simulink model "SPMSM_speed_control_with_decoupling"  (R2023b)
settings: Solver=ode45  StartTime=0.0  StopTime=3  MaxStep=0.001  RelTol=1e-3
values from neighbouring files (symbols this model uses):
  J_motor = 0.0027    [PMSM_parameter2.m]
  Lamda = 0.1194    [PMSM_parameter2.m]
  Ld = 0.0003752    [PMSM_parameter2.m]
  Lq = 0.0003752    [PMSM_parameter2.m]
  Ls = 0.0003752    [PMSM_parameter2.m]
  Pole = 2    [PMSM_parameter2.m]
  R = 0.2    [PMSM_parameter2.m]
  T_load = 10    [PMSM_parameter2.m]
  w_base = (60/(2*pi))*(v_rated/sqrt((Ls^2)*(T_load/1.5*Pole*Lamda)^2+(Lamda^2)))    [PMSM_parameter2.m]
  w_ref = 3000    [PMSM_parameter2.m]
undefined symbols (not defined in the file or in its folder): v_rated
libraries: mcbcontrolslib x2, simulink_extras x1, slpidlib x1
settings Model: Creator=chayutht  LastModifiedBy=chayutht

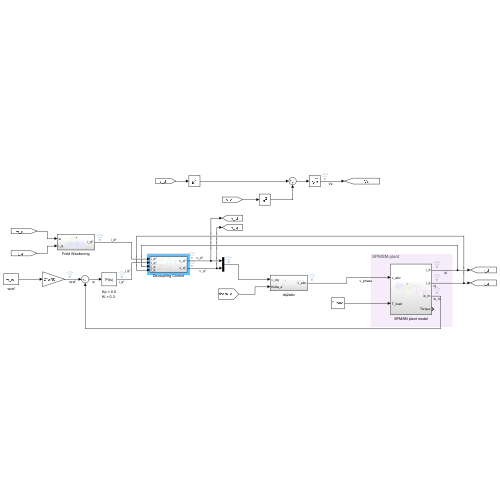
[thumbnail: Simulink's stored preview of the top-level diagram]
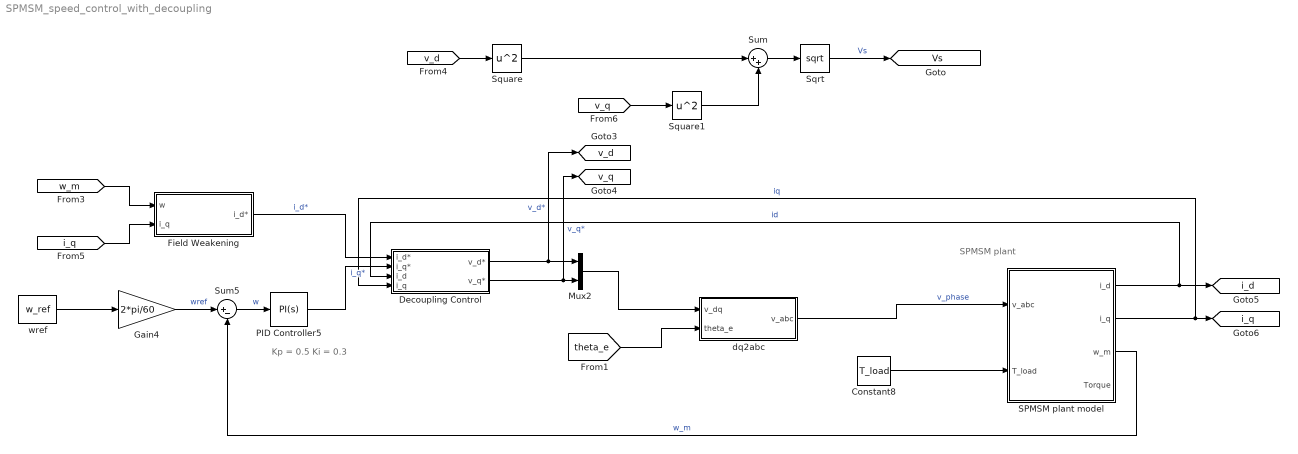
== system SPMSM_speed_control_with_decoupling ==
  note: SPMSM plant
  note: Kp = 0.5
      | Ki = 0.3
  Constant8 : Constant  Value=T_load
  Decoupling Control : Subsystem
  Field Weakening : Subsystem
  Gain4 : Gain  Gain=2*pi/60
  Mux2 : Mux  Inputs=2
  PID Controller5 : slpidlib/PID Controller  Controller=PI  Form=Parallel  TimeDomain=Continuous-time  UseExternalTs=off  SampleTime=-1  IntegratorMethod=Forward Euler  FilterMethod=Forward Euler  ControllerParametersSource=internal  P=0.2  I=0.3  UseKiTs=off  D=0  N=100  UseFilter=on  TunerSelectOption=Transfer Function Based (PID Tuner App)  InitialConditionSource=internal  InitialConditionForIntegrator=0  InitialConditionForFilter=0  DifferentiatorICPrevScaledInput=0  ExternalReset=none  TrackingMode=off  Kt=1  LimitOutput=off  SatLimitsSource=internal  UpperSaturationLimit=inf  LowerSaturationLimit=-inf  LinearizeAsGain=on  AntiWindupMode=none  Kb=1  LimitIntegrator=off  UpperIntegratorSaturationLimit=inf  LowerIntegratorSaturationLimit=-inf  POutMin=[]  POutMax=[]  IOutMin=[]  IOutMax=[]  DOutMin=[]  DOutMax=[]  NOutMin=[]  NOutMax=[]  SumOutMin=[]  SumOutMax=[]  SaturationOutMin=[]  SaturationOutMax=[]  PParamMin=[]  PParamMax=[]  IParamMin=[]  IParamMax=[]  DParamMin=[]  DParamMax=[]  NParamMin=[]  NParamMax=[]  KbParamMin=[]  KbParamMax=[]  KtParamMin=[]  KtParamMax=[]  KbOutMin=[]  KbOutMax=[]  KtOutMin=[]  KtOutMax=[]  IntegratorOutMin=[]  IntegratorOutMax=[]  FilterOutMin=[]  FilterOutMax=[]  SumI1OutMin=[]  SumI1OutMax=[]  SumI2OutMin=[]  SumI2OutMax=[]  SumI3OutMin=[]  SumI3OutMax=[]  SumI4OutMin=[]  SumI4OutMax=[]  SumDOutMin=[]  SumDOutMax=[]  DifferentiatorOutMin=[]  DifferentiatorOutMax=[]  FilterDiffOutCoefMin=[]  FilterDiffOutCoefMax=[]  ReciprocalOutMin=[]  ReciprocalOutMax=[]  SumDenOutMin=[]  SumDenOutMax=[]  SumNumOutMin=[]  SumNumOutMax=[]  DivideOutMin=[]  DivideOutMax=[]  UdiffTsProdOutMin=[]  UdiffTsProdOutMax=[]  NTsProdOutMin=[]  NTsProdOutMax=[]  UintegralTsProdOutMin=[]  UintegralTsProdOutMax=[]  UngainTsProdOutMin=[]  UngainTsProdOutMax=[]  ClampingZeroOutDataTypeStr=Inherit: Inherit via back propagation  ClampingZeroOutMin=[]  ClampingZeroOutMax=[]  FilterDenConstantOutDataTypeStr=Inherit: Inherit via back propagation  FilterDenConstantOutMin=[]  FilterDenConstantOutMax=[]  PCopyOutDataTypeStr=Inherit: Inherit via back propagation  PCopyOutMin=[]  PCopyOutMax=[]  NCopyOutDataTypeStr=Inherit: Inherit via back propagation  NCopyOutMin=[]  NCopyOutMax=[]  IntegratorContinuousStateAttributes=''  IntegratorStateMustResolveToSignalObject=off  IntegratorRTWStateStorageClass=Auto  FilterContinuousStateAttributes=''  FilterStateMustResolveToSignalObject=off  FilterRTWStateStorageClass=Auto  ParallelPVariant=InternalParameters  IdealPVariant=Disabled  IVariant=InternalParameters  DVariant=Disabled  IntegratorVariant=Continuous  SatVariant=Disabled  AWVariant=Passthrough  PCopyVariant=Disabled  TRVariant=Disabled  FdbkBlocksVariant=Forward  IdealPFdbkVariant=Disabled  SatFdbkVariant=Disabled  DerivativeFilterVariant=Disabled  NVariant=Disabled  NCopyVariant=Disabled_SignalSpec  FilterICVariant=Disabled  IntegratorICVariant=InternalICs  ExternalResetVariant=Disabled  TRSumVariant=Passthrough  SumFdbkVariant=Disabled  SumVariant=Sum_PI  TsampFilterVariant=InternalTs  TsampNgainVariant=Passthrough  TsampIntegralVariant=Disabled_SignalSpec  ExternalSaturationOutDataTypeStr=Inherit: Same as second input
  SPMSM plant model : Subsystem
  Sqrt : Sqrt
  Square : Math  Operator=square
  Square1 : Math  Operator=square
  Sum : Sum  Inputs=|++
  Sum5 : Sum  Inputs=|+-
  dq2abc : Subsystem
  wref : Constant  Value=w_ref
  tag scope: Vs=global, i_d=global, i_q=global, v_d=global, v_q=global
  wires:
  [w_m] -> Field Weakening/1(w)
  PID Controller5/1 -> Decoupling Control/2(i_q*)  "i_q*"
  Gain4/1 -> Sum5/1  "wref"
  Decoupling Control/1(v_d*) -> [v_d], Mux2/1  "v_d*"
  Mux2/1 -> dq2abc/1(v_dq)
  [i_q] -> Field Weakening/2(i_q)
  Sum5/1 -> PID Controller5/1  "w"
  SPMSM plant model/1(i_d) -> Decoupling Control/3(i_d), [i_d]  "id"
  dq2abc/1(v_abc) -> SPMSM plant model/1(v_abc)  "v_phase"
  wref/1 -> Gain4/1
  Decoupling Control/2(v_q*) -> [v_q], Mux2/2  "v_q*"
  Field Weakening/1(i_d*) -> Decoupling Control/1(i_d*)  "i_d*"
  [theta_e] -> dq2abc/2(theta_e)
  SPMSM plant model/3(w_m) -> Sum5/2  "w_m"
  Constant8/1 -> SPMSM plant model/2(T_load)
  SPMSM plant model/2(i_q) -> Decoupling Control/4(i_q), [i_q]  "iq"
  Sum/1 -> Sqrt/1
  Sqrt/1 -> [Vs]  "Vs"
  Square/1 -> Sum/1
  [v_d] -> Square/1
  Square1/1 -> Sum/2
  [v_q] -> Square1/1

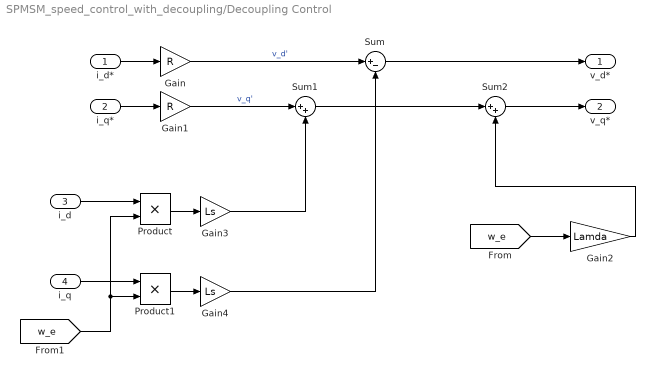
== system SPMSM_speed_control_with_decoupling/Decoupling Control ==
  i_d* : Inport
  i_q* : Inport  Port=2
  i_d : Inport  Port=3
  i_q : Inport  Port=4
  Gain : Gain  Gain=R
  Gain1 : Gain  Gain=R
  Gain2 : Gain  Gain=Lamda
  Gain3 : Gain  Gain=Ls
  Gain4 : Gain  Gain=Ls
  Product : Product
  Product1 : Product
  Sum : Sum  Inputs=|+-
  Sum1 : Sum  Inputs=|++
  Sum2 : Sum  Inputs=|++
  v_d* : Outport
  v_q* : Outport  Port=2
  wires:
  i_d*/1 -> Gain/1
  i_q*/1 -> Gain1/1
  Gain1/1 -> Sum1/1  "v_q'"
  Gain/1 -> Sum/1  "v_d'"
  Sum1/1 -> Sum2/1
  Sum2/1 -> v_q*/1
  Sum/1 -> v_d*/1
  [w_e] -> Gain2/1
  Gain2/1 -> Sum2/2
  i_d/1 -> Product/1
  [w_e] -> Product1/2, Product/2
  i_q/1 -> Product1/1
  Product/1 -> Gain3/1
  Product1/1 -> Gain4/1
  Gain3/1 -> Sum1/2
  Gain4/1 -> Sum/2

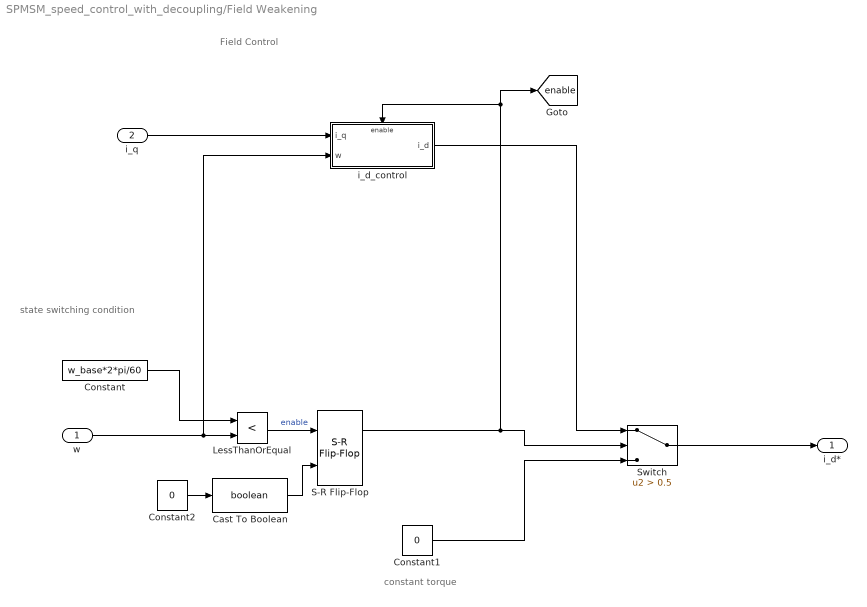
== system SPMSM_speed_control_with_decoupling/Field Weakening ==
  note: Field Control
  note: state switching condition
  note: constant torque
  w : Inport
  i_q : Inport  Port=2
  Cast To Boolean : DataTypeConversion  OutDataTypeStr=boolean  SaturateOnIntegerOverflow=off  RndMeth=Floor
  Constant : Constant  Value=w_base*2*pi/60
  Constant1 : Constant  Value=0
  Constant2 : Constant  Value=0
  LessThanOrEqual : RelationalOperator  Operator=<  OutDataTypeStr=boolean  RndMeth=Simplest  InputSameDT=off
  S-R Flip-Flop : simulink_extras/Flip Flops/S-R Flip-Flop  initial_condition=0
  Switch : Switch  Criteria=u2 > Threshold  Threshold=0.5  SaturateOnIntegerOverflow=off  InputSameDT=off
  i_d_control : Subsystem
  i_d* : Outport
  tag scope: enable=global
  wires:
  Constant/1 -> LessThanOrEqual/1
  LessThanOrEqual/1 -> S-R Flip-Flop/1  "enable"
  w/1 -> LessThanOrEqual/2, i_d_control/2(w)
  S-R Flip-Flop/1 -> Switch/2, [enable], i_d_control/Enable
  Constant1/1 -> Switch/3
  Constant2/1 -> Cast To Boolean/1
  Switch/1 -> i_d*/1
  i_q/1 -> i_d_control/1(i_q)
  i_d_control/1(i_d) -> Switch/1
  Cast To Boolean/1 -> S-R Flip-Flop/2

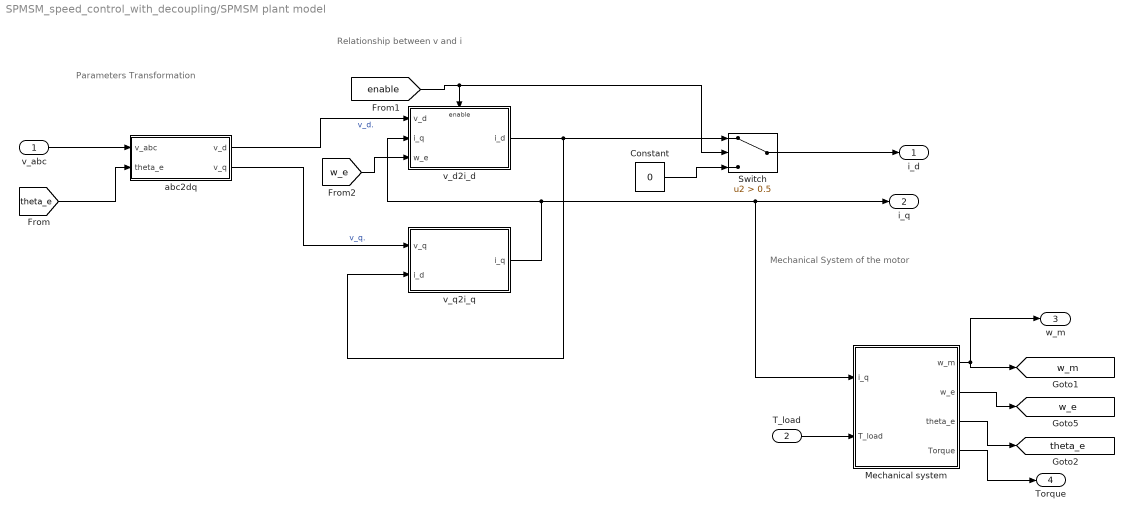
== system SPMSM_speed_control_with_decoupling/SPMSM plant model ==
  note: Mechanical System of the motor
  note: Relationship between v and i
  note: Parameters Transformation
  v_abc : Inport
  T_load : Inport  Port=2
  Constant : Constant  Value=0
  Mechanical system : Subsystem
  Switch : Switch  Criteria=u2 > Threshold  Threshold=0.5  SaturateOnIntegerOverflow=off  InputSameDT=off
  abc2dq : Subsystem
  v_d2i_d : Subsystem
  v_q2i_q : Subsystem
  i_d : Outport
  i_q : Outport  Port=2
  w_m : Outport  Port=3
  Torque : Outport  Port=4
  tag scope: theta_e=global, w_e=global, w_m=global
  wires:
  v_abc/1 -> abc2dq/1(v_abc)
  abc2dq/2(v_q) -> v_q2i_q/1(v_q)  "v_q."
  [theta_e] -> abc2dq/2(theta_e)
  T_load/1 -> Mechanical system/2(T_load)
  abc2dq/1(v_d) -> v_d2i_d/1(v_d)  "v_d."
  v_d2i_d/1(i_d) -> Switch/1, v_q2i_q/2(i_d)
  v_q2i_q/1(i_q) -> v_d2i_d/2(i_q), i_q/1, Mechanical system/1(i_q)
  Mechanical system/1(w_m) -> [w_m], w_m/1
  Mechanical system/3(theta_e) -> [theta_e]
  Mechanical system/2(w_e) -> [w_e]
  Mechanical system/4(Torque) -> Torque/1
  [enable] -> Switch/2, v_d2i_d/Enable
  Constant/1 -> Switch/3
  Switch/1 -> i_d/1
  [w_e] -> v_d2i_d/3(w_e)

== system SPMSM_speed_control_with_decoupling/dq2abc ==
  note: Inverse Park Transform
  note: Inverse Clark Transform
  v_dq : Inport
  theta_e : Inport  Port=2
  Demux : Demux  Outputs=2
  Mux : Mux  Inputs=3
  Sine-Cosine Lookup1 : mcbcontrolslib/Sine-Cosine Lookup  AngleInput=Radians  N_points=1024
      settings: LibrarySourceBlock=mcblib/Controls/Math Transforms/Sine-Cosine Lookup
  dq2xy : Subsystem
  xy2abc : Subsystem
  v_abc : Outport
  wires:
  theta_e/1 -> Sine-Cosine Lookup1/1
  Sine-Cosine Lookup1/1 -> dq2xy/3(sin_theta)  "sin"
  Sine-Cosine Lookup1/2 -> dq2xy/4(cos_theta)  "cos"
  v_dq/1 -> Demux/1
  Demux/1 -> dq2xy/1(v_d)  "v_d"
  Demux/2 -> dq2xy/2(v_q)  "v_q"
  dq2xy/1(v_xy) -> xy2abc/1(v_xy)  "v_x"
  xy2abc/2(v_b) -> Mux/2
  xy2abc/3(v_c) -> Mux/3
  xy2abc/1(v_a) -> Mux/1
  Mux/1 -> v_abc/1  "v_abc"

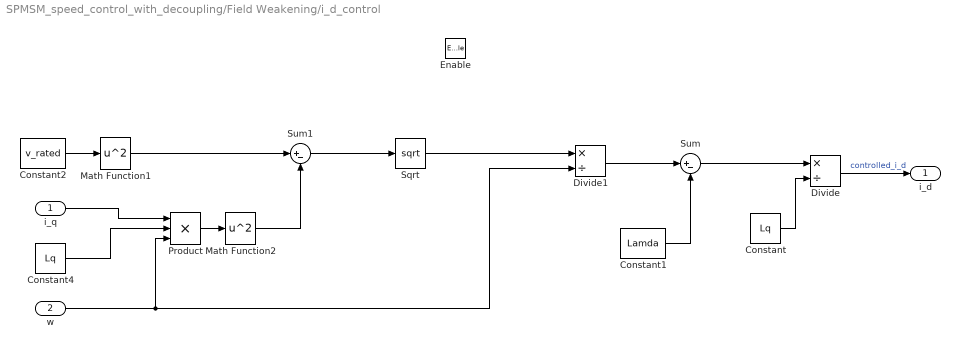
== system SPMSM_speed_control_with_decoupling/Field Weakening/i_d_control ==
  i_q : Inport
  w : Inport  Port=2
  Enable : EnablePort
  Constant : Constant  Value=Lq
  Constant1 : Constant  Value=Lamda
  Constant2 : Constant  Value=v_rated
  Constant4 : Constant  Value=Lq
  Divide : Product  Inputs=*/
  Divide1 : Product  Inputs=*/
  Math Function1 : Math  Operator=square
  Math Function2 : Math  Operator=square
  Product : Product  Inputs=3
  Sqrt : Sqrt
  Sum : Sum  Inputs=|+-
  Sum1 : Sum  Inputs=|+-
  i_d : Outport
  wires:
  Divide/1 -> i_d/1  "controlled_i_d"
  Constant/1 -> Divide/2
  Sum/1 -> Divide/1
  Constant1/1 -> Sum/2
  Divide1/1 -> Sum/1
  w/1 -> Product/3, Divide1/2
  Sqrt/1 -> Divide1/1
  Sum1/1 -> Sqrt/1
  Math Function1/1 -> Sum1/1
  Product/1 -> Math Function2/1
  Math Function2/1 -> Sum1/2
  Constant4/1 -> Product/2
  i_q/1 -> Product/1
  Constant2/1 -> Math Function1/1

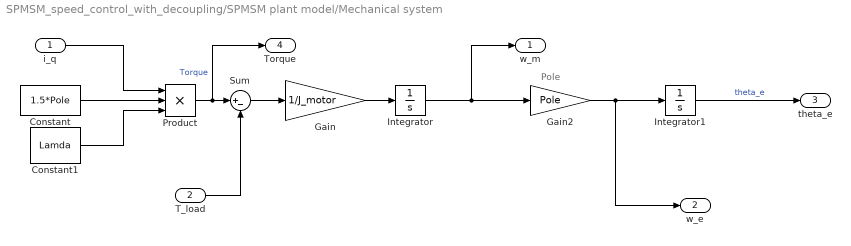
== system SPMSM_speed_control_with_decoupling/SPMSM plant model/Mechanical system ==
  note: Pole
  i_q : Inport
  T_load : Inport  Port=2
  Constant : Constant  Value=1.5*Pole
  Constant1 : Constant  Value=Lamda
  Gain : Gain  Gain=1/J_motor
  Gain2 : Gain  Gain=Pole
  Integrator : Integrator
  Integrator1 : Integrator
  Product : Product  Inputs=***
  Sum : Sum  Inputs=|+-
  w_m : Outport
  w_e : Outport  Port=2
  theta_e : Outport  Port=3
  Torque : Outport  Port=4
  wires:
  Product/1 -> Torque/1, Sum/1  "Torque"
  Gain2/1 -> Integrator1/1, w_e/1
  Constant1/1 -> Product/3
  Constant/1 -> Product/2
  Integrator/1 -> Gain2/1, w_m/1
  Sum/1 -> Gain/1
  Integrator1/1 -> theta_e/1  "theta_e"
  Gain/1 -> Integrator/1
  i_q/1 -> Product/1
  T_load/1 -> Sum/2

== system SPMSM_speed_control_with_decoupling/SPMSM plant model/abc2dq ==
  v_abc : Inport
  theta_e : Inport  Port=2
  *sqrt(2/3) : Gain  Gain=sqrt(2/3)  Multiplication=Matrix(K*u)
  Clark Transform : Subsystem
  Demux : Demux  Outputs=2
  Demux1 : Demux  Outputs=3
  Park Transform : Subsystem
  Sine-Cosine Lookup4 : mcbcontrolslib/Sine-Cosine Lookup  AngleInput=Radians  N_points=1024
      settings: LibrarySourceBlock=mcblib/Controls/Math Transforms/Sine-Cosine Lookup
  v_d : Outport
  v_q : Outport  Port=2
  wires:
  v_abc/1 -> *sqrt(2/3)/1
  Demux1/1 -> Clark Transform/1(v_a)
  Demux1/2 -> Clark Transform/2(v_b)
  Demux1/3 -> Clark Transform/3(v_c)
  *sqrt(2/3)/1 -> Demux1/1
  Clark Transform/1(v_xy) -> Park Transform/1(v_xy)  "v_xy"
  Park Transform/1(v_dq) -> Demux/1
  Demux/1 -> v_d/1  "v_d"
  Demux/2 -> v_q/1  "v_q"
  Sine-Cosine Lookup4/1 -> Park Transform/2(sin_theta)  "sin"
  theta_e/1 -> Sine-Cosine Lookup4/1
  Sine-Cosine Lookup4/2 -> Park Transform/3(cos_theta)  "cos"

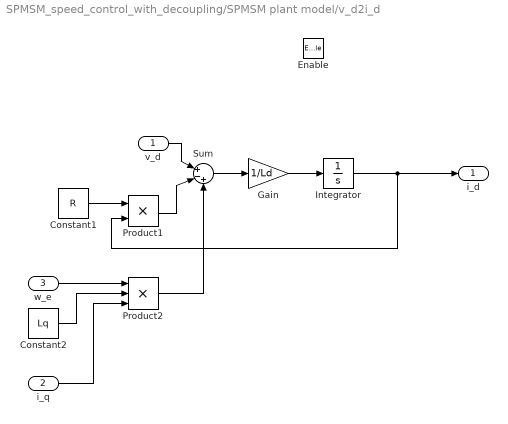
== system SPMSM_speed_control_with_decoupling/SPMSM plant model/v_d2i_d ==
  v_d : Inport
  i_q : Inport  Port=2
  w_e : Inport  Port=3
  Enable : EnablePort
  Constant1 : Constant  Value=R
  Constant2 : Constant  Value=Lq
  Gain : Gain  Gain=1/Ld
  Integrator : Integrator
  Product1 : Product  Inputs=**
  Product2 : Product  Inputs=***
  Sum : Sum  Inputs=|+-+
  i_d : Outport
  wires:
  Sum/1 -> Gain/1
  i_q/1 -> Product2/3
  v_d/1 -> Sum/1
  Gain/1 -> Integrator/1
  Constant1/1 -> Product1/1
  Product1/1 -> Sum/2
  Constant2/1 -> Product2/2
  Product2/1 -> Sum/3
  Integrator/1 -> i_d/1, Product1/2
  w_e/1 -> Product2/1

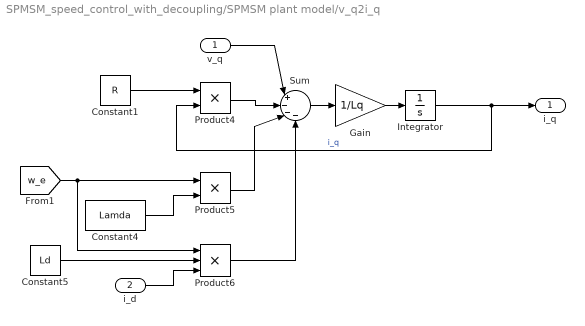
== system SPMSM_speed_control_with_decoupling/SPMSM plant model/v_q2i_q ==
  v_q : Inport
  i_d : Inport  Port=2
  Constant1 : Constant  Value=R
  Constant4 : Constant  Value=Lamda
  Constant5 : Constant  Value=Ld
  Gain : Gain  Gain=1/Lq
  Integrator : Integrator
  Product4 : Product  Inputs=**
  Product5 : Product  Inputs=**
  Product6 : Product  Inputs=***
  Sum : Sum  Inputs=|+---
  i_q : Outport
  wires:
  Integrator/1 -> Product4/2, i_q/1  "i_q"
  Sum/1 -> Gain/1
  v_q/1 -> Sum/1
  Constant1/1 -> Product4/1
  Gain/1 -> Integrator/1
  Product4/1 -> Sum/2
  [w_e] -> Product6/1, Product5/1
  Constant4/1 -> Product5/2
  Product5/1 -> Sum/3
  Product6/1 -> Sum/4
  Constant5/1 -> Product6/2
  i_d/1 -> Product6/3

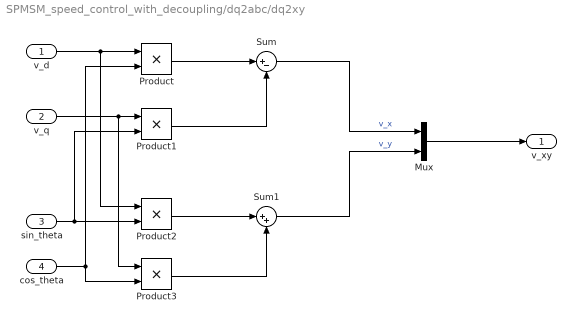
== system SPMSM_speed_control_with_decoupling/dq2abc/dq2xy ==
  v_d : Inport
  v_q : Inport  Port=2
  sin_theta : Inport  Port=3
  cos_theta : Inport  Port=4
  Mux : Mux  Inputs=2
  Product{,1..3} (4 alike) : Product
  Sum : Sum  Inputs=|+-
  Sum1 : Sum  Inputs=|++
  v_xy : Outport
  wires:
  v_d/1 -> Product2/1, Product/1
  cos_theta/1 -> Product/2, Product3/2
  v_q/1 -> Product3/1, Product1/1
  sin_theta/1 -> Product2/2, Product1/2
  Product/1 -> Sum/1
  Product1/1 -> Sum/2
  Sum/1 -> Mux/1  "v_x"
  Product2/1 -> Sum1/1
  Product3/1 -> Sum1/2
  Sum1/1 -> Mux/2  "v_y"
  Mux/1 -> v_xy/1

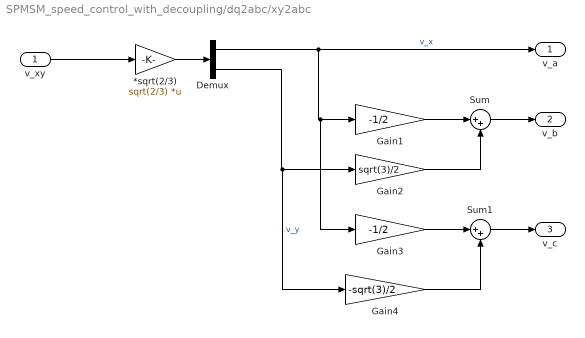
== system SPMSM_speed_control_with_decoupling/dq2abc/xy2abc ==
  v_xy : Inport
  *sqrt(2/3) : Gain  Gain=sqrt(2/3)  Multiplication=Matrix(K*u)
  Demux : Demux  Outputs=2
  Gain1 : Gain  Gain=-1/2
  Gain2 : Gain  Gain=sqrt(3)/2
  Gain3 : Gain  Gain=-1/2
  Gain4 : Gain  Gain=-sqrt(3)/2
  Sum : Sum  Inputs=|++
  Sum1 : Sum  Inputs=|++
  v_a : Outport
  v_b : Outport  Port=2
  v_c : Outport  Port=3
  wires:
  v_xy/1 -> *sqrt(2/3)/1
  Demux/1 -> Gain3/1, Gain1/1, v_a/1  "v_x"
  Demux/2 -> Gain4/1, Gain2/1  "v_y"
  Sum/1 -> v_b/1
  Gain1/1 -> Sum/1
  Gain2/1 -> Sum/2
  Sum1/1 -> v_c/1
  Gain4/1 -> Sum1/2
  Gain3/1 -> Sum1/1
  *sqrt(2/3)/1 -> Demux/1

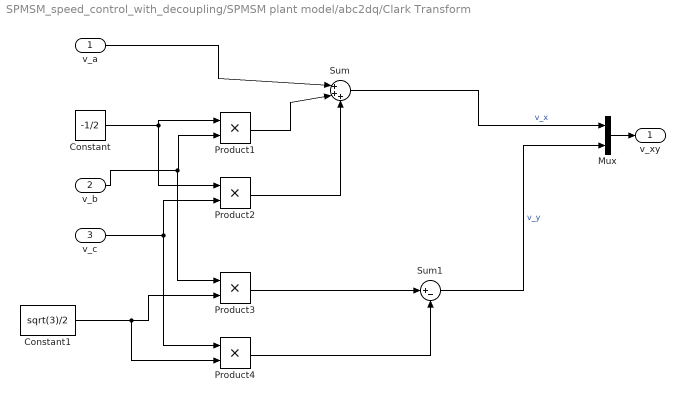
== system SPMSM_speed_control_with_decoupling/SPMSM plant model/abc2dq/Clark Transform ==
  v_a : Inport
  v_b : Inport  Port=2
  v_c : Inport  Port=3
  Constant : Constant  Value=-1/2
  Constant1 : Constant  Value=sqrt(3)/2
  Mux : Mux  Inputs=2
  Product{1..4} (4 alike) : Product
  Sum : Sum  Inputs=|+++
  Sum1 : Sum  Inputs=|+-
  v_xy : Outport
  wires:
  v_a/1 -> Sum/1
  Constant/1 -> Product1/1, Product2/1
  v_b/1 -> Product3/1, Product1/2
  Product1/1 -> Sum/2
  v_c/1 -> Product4/1, Product2/2
  Product2/1 -> Sum/3
  Constant1/1 -> Product4/2, Product3/2
  Product3/1 -> Sum1/1
  Product4/1 -> Sum1/2
  Mux/1 -> v_xy/1
  Sum/1 -> Mux/1  "v_x"
  Sum1/1 -> Mux/2  "v_y"

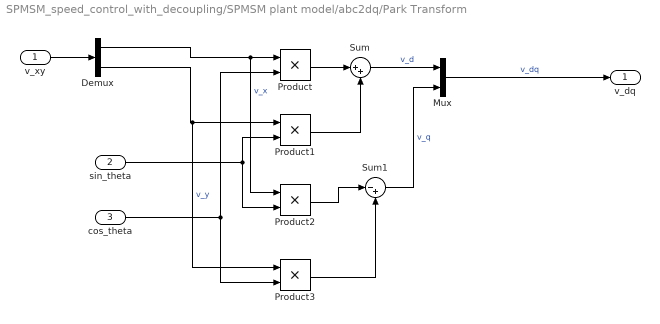
== system SPMSM_speed_control_with_decoupling/SPMSM plant model/abc2dq/Park Transform ==
  v_xy : Inport
  sin_theta : Inport  Port=2
  cos_theta : Inport  Port=3
  Demux : Demux  Outputs=2
  Mux : Mux  Inputs=2
  Product{,1..3} (4 alike) : Product
  Sum : Sum  Inputs=|++
  Sum1 : Sum  Inputs=|-+
  v_dq : Outport
  wires:
  v_xy/1 -> Demux/1
  Demux/1 -> Product/1, Product2/1  "v_x"
  Demux/2 -> Product3/1, Product1/1  "v_y"
  cos_theta/1 -> Product3/2, Product/2
  sin_theta/1 -> Product2/2, Product1/2
  Product/1 -> Sum/1
  Product1/1 -> Sum/2
  Sum/1 -> Mux/1  "v_d"
  Product2/1 -> Sum1/1
  Product3/1 -> Sum1/2
  Sum1/1 -> Mux/2  "v_q"
  Mux/1 -> v_dq/1  "v_dq"
